simulink model "FDIA_21_TRAINING"  (R2021a)
settings: Solver=ode113  StartTime=0.0  StopTime=20  RelTol=1e-3
undefined symbols (not defined in the file or in its folder): Discrete, linsys1, Time
libraries: spsThreePhaseVIMeasurementLib x46, spsThreePhasePISectionLineLib x20, spsThreePhaseSeriesRLCLoadLib x12, simulink x6, spsThreePhaseTransformerTwoWindingsLib x5, spsThreePhaseBreakerLib x5, ctrlSharedLib x3, spsThreePhaseDynamicLoadLib x3, spsSynchronousMachinepuStandardLib x3, spsThreePhaseParallelRLCLoadLib x3, spsExcitationSystemLib x3, spsGenericPowerSystemStabilizerLib x3
(part 1 of 3)
settings Model: Creator=root  LastModifiedBy=suman
settings DataIOCC: SaveFormat=Array  SaveOutput=off  SignalLogging=off  DSMLogging=off  SaveTime=off  ReturnWorkspaceOutputs=off
settings DebuggingCC: SFMachineParentedDataDiag=warning  ArithmeticOperatorsInVariantConditions=warning
settings SFSimCC: CustomCodeUndefinedFunction=UseInterfaceOnly

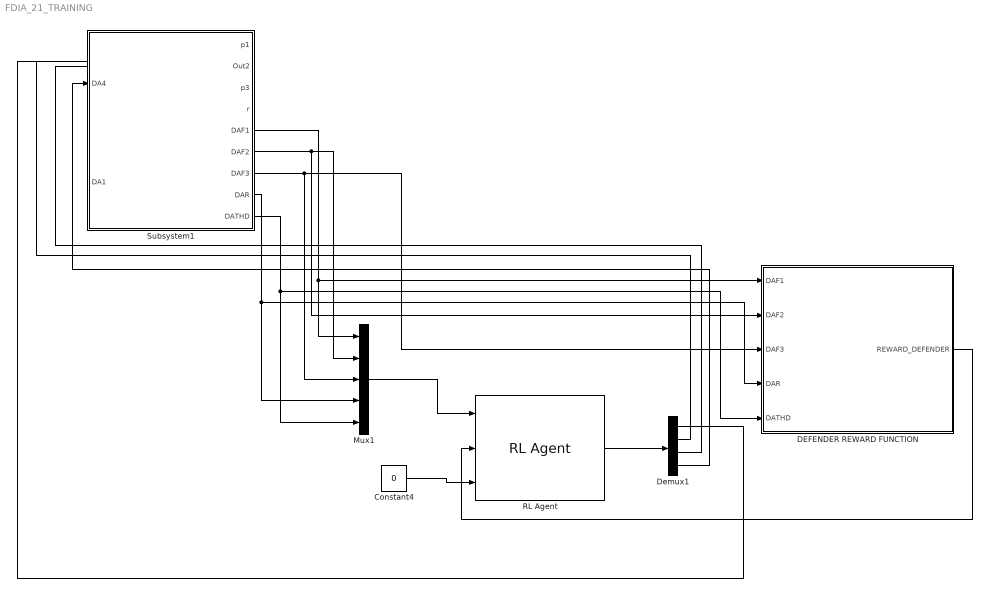
== system FDIA_21_TRAINING ==
  Constant4 : Constant  Value=0
  DEFENDER REWARD FUNCTION : MATLAB Function  TreatAsAtomicUnit=on
  Demux1 : Demux
  Mux1 : Mux  Inputs=5
  RL Agent : rllib/RL Agent  Agent=agentFDIA14  ExternalActionAsInput=off  ProvideCumRwd=off  TreatAsDirectFeedthrough=on
  Subsystem1 : Subsystem
  wires:
  Subsystem1/5(DAF1) -> Mux1/1, DEFENDER REWARD FUNCTION/1(DAF1)
  Subsystem1/6(DAF2) -> DEFENDER REWARD FUNCTION/2(DAF2), Mux1/2
  Subsystem1/7(DAF3) -> DEFENDER REWARD FUNCTION/3(DAF3), Mux1/3
  Subsystem1/8(DAR) -> DEFENDER REWARD FUNCTION/4(DAR), Mux1/4
  Subsystem1/9(DATHD) -> DEFENDER REWARD FUNCTION/5(DATHD), Mux1/5
  Mux1/1 -> RL Agent/1
  Constant4/1 -> RL Agent/3
  Demux1/1 -> ?
  Demux1/2 -> ?
  Demux1/3 -> ?
  Demux1/4 -> Subsystem1/1(DA4)
  RL Agent/1 -> Demux1/1
  DEFENDER REWARD FUNCTION/1(REWARD_DEFENDER) -> RL Agent/2
